simulink model "RB_KAIROS_ArmOnly"  (R2020b)
(part 10 of 17)

-t16229+t16408+t16412+t16445-q5d.*(t3933+t3938+t3951+t4005+t4112+t4113+t4134+t4154+t4229+t4246+t4307+t4325+t4454+t4458+t4463+t4523+t5038+t5089+t5148+t5157+t5202+t5353+t5381+t5473+t5512+t5567+t5662+t6241+t6342+t6347+t6369+t6562+t6652+t6708+t6712+t6714+t6723+t6752+t6768+t6769+t6919+t7058+t7523+t7596+t7597+t7609+t7679+t7722+t7742+t7760+t7905+t7947+t7988+t8037+t8059+t8078+t8196+t8425+t8443+t8446+t8662+t8680+t8736+t8748+t8773+t9037+t9039+t9294-t9304-t9351+t9539-t9543+t9575+t9587+t9607+t9692+t9697+t10370+t10493+t10503-t10576+t10667+t11245+t11261-t11450-t11460+t11665+t12004+t12081+t12087+t12282+t12284+(t5329.*(t2740+t3849+t3968+t3972-t5255+t17.*(t260+t468+t570+t2298).*7.35522e-1))./4.0+(t5441.*(-t1476-t1540+t2091+t2165+t2579+t8.*(t260+t468+t570+t2298)))./4.0+(t5345.*(-t3823+t3970+t5243+t9.*(t260+t468+t570+t2298).*7.35522e-1+t972.*(t71-t391)+t2777.*(t71-t391)))./4.0+(t6046.*(t1492+t2158+t2696-t4727))./4.0+(t4024.*(t3063+t3528+t3966-t5230))./4.0+(t3780.*(-t3045-t3218+t3458+t3539+t3878+t8.*(t260+t468+t570+t2298).*1.666555))./4.0+(t7796.*(t824+t2543+t2699+t2707-t4767+t17.*(t260+t468+t570+t2298)))./4.0+(t7797.*(-t2550+t2696+t2698+t4771+t9.*(t260+t468+t570+t2298)+t147.*(t71-t391)))./4.0)+q7d.*t16166-q3d.*t16340-q2d.*t16358+q4d.*(t3271+t3297+t3326+t3353+t3802+t3910+t3985+t4882+t5261+t5276+t5573+t5623+t6440+t6631+t6672+t6688+t6739+t6751+t8140+t8209+t8318+t13.*t35.*9.119126684115e-2+t13.*t42.*1.02650375589525e-1+t7.*t5928.*2.11820788799e-1+t15.*t5999.*2.11820788799e-1+t7.*t8044.*1.727815e-1+t15.*t8065.*1.727815e-1-(t4774.*t5331)./2.0-(t5443.*t7080)./2.0+(t4021.*t8709)./2.0-(t4024.*t8713)./2.0-(t6046.*t6744)./2.0+(t6069.*t6729)./2.0-(t3752.*t9104)./2.0+(t5696.*t10096)./2.0-(t5329.*t10753)./2.0-(t5345.*t10763)./2.0+(t8433.*t8477)./2.0-(t7796.*t9187)./2.0-(t7797.*t9197)./2.0+(t3424.*(t985+t3399-t13.*t42.*1.01140545e-1-t7.*t223.*5.034347249e-2))./2.0)-q6d.*(t4397+t4399+t4408+t4414+t4416+t4433+t4468+t4826+t4836+t4935+t4950-t5074+t5086+t5338+t5379+t5403+t5811+t5893+t6326+t6378+t6416+t6528+t6532+t6575+t7027+t7140+t7189+t7610+t7619+t8005+t8150+t8580+t8645+t8663+t8691+t8880+t9199+t9283+t9291+t9324+t9330+t9544+t9558-t9714+t9742-t9840+t10186+t10200+t10440+t10525-t10672+t10841+t10889-t10894+t10907+t11004+t11007+t11123+t11136+t11573+t11639+t11643+t12089+t12096+t8.*(t295-t13.*t42.*(3.3e+1./4.0e+2)).*5.01208083475e-2+t16.*(t295-t13.*t42.*(3.3e+1./4.0e+2)).*1.17633784675e-2),-t16190+t16359-t16361+t16365+phid.*(t2261+t2304+t2384+t3146+t3288+t3303+t3305+t3351+t3740+t4007+t4025+t4048+t4164+t4320+t4571+t4863+t4946+t4985+t5104+t5114+t5279+t5328+t5355+t5375+t5406+t5629+t5632+t5645+t5747+t5771+t5790+t5808+t5825+t5907+t5980+t6061+t6136+t6292+t6454+t6571+t6648+t6666+t6668+t6700+t6760+t6829+t6891+t6895+t6922+t7006+t7013+t7091+t7110+t7291+t7340+t7554+t7564+t7566+t7626+t7664+t7825+t7850+t7986+t8001+t8122+t8346+t8375+t8385+t8598+t8639+t8649+t8684+t8718+t8737+t8827+t8959+t9105+t10453+t10686-t10825-t10829-t10978+t10993-t11184+t11191+t11263+t11287-t11408-t11418+t11513-t11868+t11980+t12150+t12196+t12202+t12209-t12308-t12319-t12380-t12390-t12406+t12759+t12934+t13157-t13262-t13275+t13449+t13471-t13579-t13588+t13670+t13684+t13978+t14042-t14159+t14166+t14221-t14225+t14226+t14262-t14635-t14682-t14726-t14727-t14762-t14764+t15126+t15130+t15176+t15180+t15488+t15489+t15494+t15495+(t7987.*(t3418-t3879+t4324+t11855+t9.*(t71-t391).*4.5305948634e-2+t17.*(t426-t581).*7.35522e-1+t9.*(t9166-t11658).*7.35522e-1))./4.0+(t7130.*(t1589-t2213-t4346+t4355+t9454+t11863+t2772.*(t71-t391)+t2775.*(t71-t391)))./4.0+(t7982.*(t3423+t3845+t3888+t3925+t4339+t9.*(t210+t2107+t7423+t9121).*7.35522e-1+t17.*(t9166-t11658).*7.35522e-1))./4.0+(t9310.*(t249-t391.*(1.1e+1./1.25e+2)-t1912.*4.252e-3+t3505+t13496+t693.*(t71-t391)+t784.*(t71-t391)))./4.0+(t9887.*(t2091+t2497+t2579+t2680+t3516+t9.*(t210+t2107+t7423+t9121)+t17.*(t9166-t11658)))./4.0+(t9896.*(t1987-t2621+t3452+t11654+t9.*(t71-t391).*6.1597e-2+t17.*(t426-t581)+t9.*(t9166-t11658)))./4.0)-q6d.*t16216-q5d.*t16260+q3d.*t16327+q7d.*(t3995+t4013+t4190+t4197+t4271+t4313+t4437+t4467+t4543+t4560+t5106+t5166-t5688+t5906+t6001-t6439+t6487+t6491+t7633+t7758-t10457-t10565+t10573+t10755-t10760-t10844+t10845-t11160+t11236-t11240+(t5837.*(t395+t9.*(t48-t349)))./4.0+(t8477.*(-t2149+t2205+t693.*(t48-t349)+t784.*(t48-t349)))./4.0+(t5696.*(t3479-t3544+t2772.*(t48-t349)+t2775.*(t48-t349)))./4.0+(t15.*t16.*(-t2182+t2241+t696.*(t48-t349)+t891.*(t48-t349)))./4.0)+q4d.*((t5443.*(-t1272-t1479+t1647+t1848+t2236))./2.0+t5.*t6.*9.119126684115e-2+t5.*t14.*1.02650375589525e-1+t6.*t13.*1.644586079438601e-3-t13.*t14.*3.9053550262761e-3-(t7.*t4531)./2.0+(t15.*t4587)./2.0+t15.*t4837.*2.11820788799e-1-t7.*t4849.*2.11820788799e-1+(t370.*t4527)./2.0-(t404.*t4534)./2.0+(t7.*t6005)./2.0-(t404.*t5810)./2.0+(t540.*t5763)./2.0-t7.*t6552.*1.727815e-1+t15.*t6546.*1.727815e-1-(t325.*t6803)./2.0+(t229.*t6983)./2.0+(t3424.*t6092)./2.0+(t4265.*t5331)./2.0+(t5952.*t6046)./2.0-(t5951.*t6069)./2.0+(t4024.*t8062)./2.0-(t4021.*t8070)./2.0-(t5696.*t9310)./2.0+(t5329.*t9896)./2.0-(t5345.*t9887)./2.0-(t7130.*t8477)./2.0-(t7797.*t7982)./2.0+(t7796.*t7987)./2.0-(t5837.*(t106-t414))./2.0+(t3752.*(t2433+t2449-t3048-t3102+t3223+t3232))./2.0-(t14.*t43.*t3173)./2.0-(t14.*t37.*t3247)./2.0+(t6.*t13.*t3321)./2.0-(t14.*t43.*t4495)./2.0-(t15.*t16.*t6029)./2.0+(t8.*t15.*t6064)./2.0-(t15.*t16.*t6917)./2.0),-t16160-t16326+t16342+t16347+t16350+t16448+q7d.*t16137-q6d.*t16180-q5d.*t16236-q4d.*(t6.*(-3.9053550262761e-3)-t14.*1.644586079438601e-3-(t14.*t3321)./2.0+t7.*t4035.*2.11820788799e-1-t15.*t4064.*2.11820788799e-1-(t7.*t4383)./2.0+(t15.*t4451)./2.0+(t228.*t4534)./2.0-(t324.*t4527)./2.0+t7.*t5635.*1.727815e-1-t15.*t5646.*1.727815e-1+(t7.*t5845)./2.0+(t228.*t5810)./2.0-(t484.*t5837)./2.0+(t325.*t6637)./2.0+(t229.*t6758)./2.0+(t4024.*t6677)./2.0-(t4021.*t6681)./2.0+(t5443.*t5543)./2.0-(t5007.*t6069)./2.0+(t5050.*t6046)./2.0+(t3752.*t7676)./2.0-(t5696.*t8547)./2.0+(t6526.*t7797)./2.0+(t6540.*t7796)./2.0+(t5329.*t9048)./2.0+(t5345.*t9049)./2.0-(t6158.*t8477)./2.0+(t5763.*(t77-t390))./2.0+(t5331.*(t923-t1076))./2.0+(t3424.*(t2812-t2860))./2.0-(t6.*t15.*t3173)./2.0-(t6.*t7.*t3247)./2.0-(t6.*t15.*t4495)./2.0-(t8.*t15.*t5877)./2.0+(t15.*t16.*t5875)./2.0+(t15.*t16.*t6704)./2.0),q7d.*t16008+q6d.*t16115+q5d.*t16125,-t16126-t16238-t16262-t16297+t16310+t16313-t16427+q7d.*t16117+q6d.*t16151,-t16116+t16182+t16218+t16246+t16273+t16276+t16377+q7d.*t16112-q5d.*t16151,-t16009+t16139+t16154+t16165-t16193+t16264-q6d.*t16112-q5d.*t16117+yd.*(t8886+t8907+t11429+t11431-t13130-t13291+t14545+t14550-t14627-t14633+t14697+t14700-t14831-t14837),q4d.*(t8804+t8829+t9145+t9354-t10997-t10998+t11097+t11101+t11270+t11284+t11370+t11376-t11511-t11517+t11533+t11535-t11550+t11836+t11844-t12393-t12803-t12903-t13160+t13243+t13244+t13328+t13331-t13538+t13926+t13928+t14116+t14121+t14584+t14754+(t5441.*(t10158+t16.*(t4542-t6448)))./4.0+(t5213.*(t10403+t9.*(t10158+t16.*(t4542-t6448)).*7.35522e-1))./4.0+(t3266.*(t5110-t6808))./4.0+(t4879.*(t4542-t6448))./4.0+(t3780.*(t10384+t16.*(t4542-t6448).*1.666555))./4.0+(t7538.*(t10174+t9.*(t10158+t16.*(t4542-t6448))))./4.0)-phid.*(t7280+t7283+t8889+t8899-t10176+t10541+t11053+t11058+t12514+t12526+t12607+t12615+t12787+t12801+t14199+t14202+t14263+t14316+t14319+t14331+t14336+t14432+t14465+t14471+t14484+t14514+t14524+t14593+t14594+t14746+t14978+t14983+t15086+t15091+t15198+t15203+t15213+t15382+t15404+t15405+t15408+t15528+t15929+t15930+t15977+t15979+t15995+t15996+t16015+t16016)-q1d.*(t7280+t7283+t8889+t8899-t10176+t10541+t11053+t11058+t11833+t11839+t12036+t12141+t12153+t12179+t12192+t12420+t12423+t12429+t12492+t12514+t12526+t12607+t12615+t12676+t12677+t12787+t12801+t12835+t12947+t12951+t13058+t13477+t13488+t13574+t13671+t13683+t13940+t14207+t14465+t14471+t14514+t14524+t14728+t14729+t14979+t14982+t15133+t15135+t15288+t15290)-q7d.*t16183-q6d.*t16232-q3d.*t16331+q2d.*(t5581+t5592-t7358-t7366+t9411+t9440+t10019+t10409+t10660+t10693+t10828+t10837+t11089+t11096+t11471+t11489+t11697+t11733+t11737+t11939+t11962+t12056+t12061+t12070+t12242+t12244+t12264+t12412+t12612+t12613+t12716+t12851+t12868+t12950+t12967+t13153+t13222+t13240+t13424+t13431+t13598+t14014+t14414+t14415+t14701+t14706+t14912+t14915+t15118+t15119)+q5d.*(t15.*(t4540+t5.*(t2425-t2468)).*1.4653732538e-2-t2726.*(t4540+t5.*(t2425-t2468))-t22.*t10153.*1.7527158935e-2-t28.*t10153.*1.7527158935e-2-t2729.*t8077-t2744.*t8077+(t3249.*t10550)./2.0+(t4884.*t10147)./2.0+(t3738.*t13362)./2.0+(t3743.*t13357)./2.0+(t5433.*t13167)./2.0+(t5434.*t13172)./2.0-t16.*t3421.*t10153.*3.67761e-1-(t16.*t10153.*(t2904-t2927))./2.0),q5d.*(t6449.*(-1.4653732538e-2)-t8225.*1.4653732538e-2-t8229.*5.034347249e-2+t2726.*t6430+(t3249.*t10586)./2.0+(t4884.*t10164)./2.0+(t3738.*t13391)./2.0+(t3743.*t13387)./2.0+(t5433.*t13182)./2.0+(t5434.*t13189)./2.0+t22.*(t6452-t8229).*1.7527158935e-2+t28.*(t6452-t8229).*1.7527158935e-2+(t16.*(t2904-t2927).*(t6452-t8229))./2.0+t16.*t3421.*(t6452-t8229).*3.67761e-1)+q3d.*(t7300-t7310-t7313-t7315+t9405+t9475+t10265+t10291+t11036+t11045+t11172+t11183+t11259+t11260+t11330-t11394+t11405+t11413-t11559+t11588+t11595+t11681+t11789+t11845+t11914+t11918+t12318+t12470+t12949+t12957+t13059+t13062+t13289+t13658+t13668+t13672+t13757+t13764+t14117+t14127+t14392+t14406+t14704+t14705+t14906+t14911+t16.*(t6472-t9256).*4.38178973375e-3+t16.*(t6847-t9563).*2.62925e-3+(t3421.*(t6834-t9565))./4.0+((t2904-t2927).*(t6472-t9256))./4.0)+phid.*t16439-q7d.*t16186-q4d.*t16312+q1d.*(t7309+t7314+t8781+t8789+t10202+t10562+t11032+t11043-t12176-t12438+t12441+t12496+t12509+t12592+t12598-t12703+t12766+t12779-t12852-t12972+t13074+t13505-t13584+t13693+t13958+t14215+t14447+t14453+t14492+t14501-t14736-t14992+t15150+t15312+((t6806-t8574).*(t921+t1317-t5853))./4.0+((t6452-t8229).*(t2810+t2988-t7937))./4.0+(t14213.*(t2740+t3849+t3968+t3972-t5255+t17.*(t260+t468+t570+t2298).*7.35522e-1))./4.0+(t13189.*(t3418-t3879+t4324-t5228+t5802+t9.*(t71-t391).*4.5305948634e-2+t17.*(t426-t581).*7.35522e-1))./4.0+(t13391.*(t1987-t2621+t3452-t4730+t5359+t9.*(t71-t391).*6.1597e-2+t17.*(t426-t581)))./4.0+(t12508.*(t1492+t2158+t2696-t4727))./4.0+(t12307.*(t3063+t3528+t3966-t5230))./4.0+(t10577.*(t495+t572+t1838+t2069+t2107))./4.0+(t10164.*(t2437+t2648+t3129+t3384+t3574))./4.0+(t5853.*(t6806-t8574))./4.0+(t6535.*(t6801-t8594))./4.0+(t7937.*(t6452-t8229))./4.0+(t8791.*(t6452-t8229))./4.0+(t14299.*(t824+t2543+t2699+t2707-t4767+t17.*(t260+t468+t570+t2298)))./4.0+t16.*t8227.*(t6452-t8229).*4.1663875e-1+(t16.*t9744.*(t6452-t8229))./4.0)+q6d.*(t10652+t11056+t11064+t12702+t12707+t12786+t12797+t12800+t12809+t12929+t12935+t13402-t13405+t13520-t13533+t14472+t14475+t14521+t14525+t16.*(t6452-t8229).*5.01208083475e-2+t16.*t3489.*(t6452-t8229).*1.838805e-1+(t16.*t5365.*(t6452-t8229))./4.0)-q2d.*(t5624+t5630+t7408+t7426+t9491+t9500+t10037+t10422+t10741+t10752+t10866+t10874+t11146+t11167-t11488+t11503+t11719+t11754-t11960+t11981+t12064+t12263+t12280+t12728+t12906+t12914+t13015+t13029-t13245-t13272-t13439-t13452-t13602-t14026+t14428+t14430+t14717+t14721+t14931-t14936+t15125-t15129+(t5634.*(t6806-t8574))./4.0+(t8050.*(t6452-t8229))./4.0+t16.*t7079.*(t6452-t8229).*4.1663875e-1+t8.*t7116.*(t6452-t8229).*4.1663875e-1+t16.*t8191.*(t6452-t8229).*1.838805e-1+(t8.*t9112.*(t6452-t8229))./4.0+(t16.*t9110.*(t6452-t8229))./4.0+(t16.*t10141.*(t6452-t8229))./4.0),t16353+t16436+q6d.*t16356-q4d.*t16425-q3d.*t16428-q2d.*t16440+q7d.*(-t4652-t4658+t4757+t4825+t5253+t5305+t5766+t5791+t7139+t7199+t7204+t8632+t8677+t8904+t9266+t12008+t12014+t12018+t14555+t14872+t15553+t15555+t15600+t15602+t15607+t15609+t15671+t15672+t8.*t11672.*3.867742437e-3+t2963.*(t71-t391)+t3167.*(t71-t391)+t4080.*(t71-t391)+t4130.*(t71-t391))+q5d.*(t4111+t4141+t4250+t4312-t4336+t4366+t4405-t4444+t5094+t5505-t5528-t6281+t6297+t7401.*1.4653732538e-2+t7552+t16.*(t1292+t2073+t2694+t11671).*8.7635794675e-3-(t5433.*(-t2550+t2696+t2698+t11659+t8.*t11672+t147.*(t71-t391)))./2.0-(t3743.*(-t3823+t3970+t11861+t8.*t11864+t972.*(t71-t391)+t2777.*(t71-t391)))./2.0-t2726.*t7344-t8.*t12392.*8.7635794675e-3-t8.*t12792.*5.2585e-3-(t3249.*t12898)./2.0+(t3421.*t13578)./2.0-(t4884.*t12266)./2.0-(t3738.*t15088)./2.0-(t5434.*t14770)./2.0+t3620.*(t71-t391)+(t12866.*(t2904-t2927))./2.0+t2729.*(-t211+t5081+t7275)+t2744.*(-t211+t5081+t7275)+t16.*(t3116+t3486+t3963+t11671.*1.666555).*5.2585e-3+(t16.*t17.*(t578.*4.28e-4+t2566-t2597+t905.*(t71-t391)+t1021.*(t71-t391)))./2.0+(t9.*t16.*(t578.*1.2516e-2+t2492-t2628+t2673+t1129.*(t71-t391)))./2.0)+q1d.*(t5882+t5909+t5994+t6543+t6782+t6854+t7120+t7165+t7889+t7975+t7991+t8042+t8045+t8246+t8535+t8621+t8894+t9066+t9109+t9364+t9383-t9580-t10145+t11824+t11834-t12218-t12604+t13210+t13216+t13321+t13323+t13464+t13483+t13613+t13614-t13817+t13833+t13834-t14019-t14020-t14105-t14106+t14637+t14692+t14806+t14903+t15020+t15022+t15067+t15071+t15367+t15396+t15650+t15666+t15836-t15838-t15844+t15845+(t9744.*(t1292+t2073+t2694+t11671))./4.0+((-t3045+t3539+t14113).*(t1492+t2158+t2696-t4727))./4.0+((-t1476+t2165+t13876).*(t3063+t3528+t3966-t5230))./4.0+((t2810+t2988-t12589).*(t495+t572+t1838+t2069+t2107))./4.0+((t921+t1317-t5853).*(t3129+t3384+t3574+t7846+t9332))./4.0+(t11470.*(-t2550+t2696+t2698+t11659+t8.*t11672+t147.*(t71-t391)))./4.0+(t10149.*(-t3823+t3970+t11861+t8.*t11864+t972.*(t71-t391)+t2777.*(t71-t391)))./4.0+(t12792.*(-t1476-t1540+t2091+t2165+t2579+t8.*(t260+t468+t570+t2298)))./4.0+(t12385.*(t2437+t2648+t3129+t3384+t3574))./4.0+(t12392.*(-t3045-t3218+t3458+t3539+t3878+t8.*(t260+t468+t570+t2298).*1.666555))./4.0+(t8227.*(t3116+t3486+t3963+t11671.*1.666555))./4.0)+yd.*(t7328+t7338+t8774+t8795+t10202+t10562+t11039+t11047+t12499+t12504+t12595+t12596+t12771+t12783+t14211+t14214+t14269+t14328+t14335+t14342+t14344+t14437+t14448+t14451+t14490+t14494+t14498+t14614+t14615+t14751+t14988+t14991+t15105+t15110+t15207+t15208+t15224+t15392+t15413+t15415+t15416+t15532+t15942+t15943+t15981+t15986+t16004+t16007+t16023+t16027),-t16207-t16368-t16433-q4d.*(t3933+t3938+t3951+t4005+t4112+t4113+t4134+t4154+t4229+t4246+t4307+t4325+t4454+t4458+t4463+t4523+t5038+t5089+t5148+t5157+t5202+t5353+t5381+t5473+t5512+t5567+t5662+t6241+t6342+t6347+t6369+t6562+t6652+t6708+t6712+t6714+t6723+t6752+t6768+t6769+t6919+t7058+t7523+t7596+t7597+t7609+t7679+t7722+t7742+t7760+t7905+t7947+t7988+t8037+t8059+t8078+t8196+t8425+t8443+t8446+t8662+t8680+t8736+t8748+t8773+t9037+t9039+t9294-t9304-t9351+t9539-t9543+t9575+t9587+t9607+t9692+t9697+t10370+t10493+t10503-t10576+t10667+t11245+t11261-t11450-t11460+t11665+t12004+t12081+t12087+t12282+t12284+(t5329.*(t2740+t3849+t3968+t3972-t5255+t17.*(t260+t468+t570+t2298).*7.35522e-1))./4.0+(t5441.*(-t1476-t1540+t2091+t2165+t2579+t8.*(t260+t468+t570+t2298)))./4.0+(t5345.*(-t3823+t3970+t5243+t9.*(t260+t468+t570+t2298).*7.35522e-1+t972.*(t71-t391)+t2777.*(t71-t391)))./4.0+(t6046.*(t1492+t2158+t2696-t4727))./4.0+(t4024.*(t3063+t3528+t3966-t5230))./4.0+(t3780.*(-t3045-t3218+t3458+t3539+t3878+t8.*(t260+t468+t570+t2298).*1.666555))./4.0+(t7796.*(t824+t2543+t2699+t2707-t4767+t17.*(t260+t468+t570+t2298)))./4.0+(t7797.*(-t2550+t2696+t2698+t4771+t9.*(t260+t468+t570+t2298)+t147.*(t71-t391)))./4.0)+q6d.*t16224-q3d.*t16316-q2d.*t16328+q7d.*(-t4652-t4658+t4757+t4825+t5253+t5305+t5687-t5698+t5766+t5791+t7139+t7199+t7204+t8632+t8677+t8904+t9266+t10330+t10589+t10591+t10853+t10861+t10967+t10977+t11455+t11823+t11832+t9.*(t260+t468+t570+t2298).*3.867742437e-3+t17.*(t260+t468+t570+t2298).*1.563719772e-3+t2963.*(t71-t391)+t3167.*(t71-t391)+t4080.*(t71-t391)+t4130.*(t71-t391))+yd.*(t7328+t7338+t8774+t8795+t10202+t10562+t11039+t11047-t12176-t12438+t12441+t12499+t12504+t12595+t12596-t12703+t12771+t12783-t12852-t12972+t13074+t13505-t13584+t13693+t13958+t14215+t14448+t14451+t14494+t14498-t14736-t14992+t15150+t15312+((t6806-t8574).*(t921+t1317-t5853))./4.0+((t6452-t8229).*(t2810+t2988-t7937))./4.0+(t14213.*(t2740+t3849+t3968+t3972-t5255+t17.*(t260+t468+t570+t2298).*7.35522e-1))./4.0+(t13189.*(t3418-t3879+t4324-t5228+t5802+t9.*(t71-t391).*4.5305948634e-2+t17.*(t426-t581).*7.35522e-1))./4.0+(t13391.*(t1987-t2621+t3452-t4730+t5359+t9.*(t71-t391).*6.1597e-2+t17.*(t426-t581)))./4.0+(t12508.*(t1492+t2158+t2696-t4727))./4.0+(t12307.*(t3063+t3528+t3966-t5230))./4.0+(t10577.*(t495+t572+t1838+t2069+t2107))./4.0+(t10164.*(t2437+t2648+t3129+t3384+t3574))./4.0+(t5853.*(t6806-t8574))./4.0+(t6535.*(t6801-t8594))./4.0+(t7937.*(t6452-t8229))./4.0+(t8791.*(t6452-t8229))./4.0+(t14299.*(t824+t2543+t2699+t2707-t4767+t17.*(t260+t468+t570+t2298)))./4.0+t16.*t8227.*(t6452-t8229).*4.1663875e-1+(t16.*t9744.*(t6452-t8229))./4.0)+q5d.*(t464.*(-5.034347249e-2)+t468.*1.4653732538e-2+t570.*1.4653732538e-2+t572.*5.034347249e-2+t4111+t4141+t4250+t4312-t4336+t4366+t4405-t4444+t5094+t5505-t5528-t6281+t6297+t7552-(t3738.*(t2740+t3849+t3968+t3972-t5255+t17.*(t260+t468+t570+t2298).*7.35522e-1))./2.0-(t3743.*(-t3823+t3970+t5243+t9.*(t260+t468+t570+t2298).*7.35522e-1+t972.*(t71-t391)+t2777.*(t71-t391)))./2.0+t16.*t6995.*8.7635794675e-3+t16.*t8600.*5.2585e-3-(t4884.*t6535)./2.0-(t3249.*t8791)./2.0+(t3421.*t10240)./2.0-t8.*(t1492+t2158+t2696-t4727).*8.7635794675e-3-t8.*(t3063+t3528+t3966-t5230).*5.2585e-3+t3620.*(t71-t391)+(t8693.*(t2904-t2927))./2.0-(t5434.*(t824+t2543+t2699+t2707-t4767+t17.*(t260+t468+t570+t2298)))./2.0-(t5433.*(-t2550+t2696+t2698+t4771+t9.*(t260+t468+t570+t2298)+t147.*(t71-t391)))./2.0+(t16.*t17.*(t578.*4.28e-4+t2566-t2597+t905.*(t71-t391)+t1021.*(t71-t391)))./2.0+(t9.*t16.*(t578.*1.2516e-2+t2492-t2628+t2673+t1129.*(t71-t391)))./2.0),t16176+t16339+t16344+t16442+q1d.*(t3806+t3818+t3974+t3983+t4108+t4155+t4171+t4184+t4245+t4316+t4343+t4431+t4439+t4766+t4803+t5368+t5520+t5548+t5627+t5717+t5768+t5770+t5792+t5799+t6059+t6157+t6266+t6389+t6426+t6429+t6557+t6564+t6945+t7035+t7143+t7203+t7211+t7375+t7592+t7616+t7706+t7711+t7812+t7816+t7843+t7906+t7924+t8200+t8257+t8359+t8409+t8611+t8625+t8664+t8726+t8901+t8924+t8965+t9004+t9192+t9308-t9352+t9672+t9676+t9883+t9900+t9927+t9937+t9938-t9969+t9990+t10015+t10281+t10347+t10366+t10516+t10717-t10751+t10788-t10805+t11029-t11060+t11104-t11133+t11302+t11310+t11411+t12001+t12003-t12356+t12404-t12460+t12490+t12812+t12813+t12938+t12940+(t8979.*(t2740+t3849+t3968+t3972-t5255+t17.*(t260+t468+t570+t2298).*7.35522e-1))./4.0+(t7646.*(-t1476-t1540+t2091+t2165+t2579+t8.*(t260+t468+t570+t2298)))./4.0+(t8981.*(-t3823+t3970+t5243+t9.*(t260+t468+t570+t2298).*7.35522e-1+t972.*(t71-t391)+t2777.*(t71-t391)))./4.0+(t9112.*(t1492+t2158+t2696-t4727))./4.0+(t7116.*(t3063+t3528+t3966-t5230))./4.0+(t6014.*(-t3045-t3218+t3458+t3539+t3878+t8.*(t260+t468+t570+t2298).*1.666555))./4.0+(t10468.*(t824+t2543+t2699+t2707-t4767+t17.*(t260+t468+t570+t2298)))./4.0+(t10469.*(-t2550+t2696+t2698+t4771+t9.*(t260+t468+t570+t2298)+t147.*(t71-t391)))./4.0)+q7d.*t16141-q6d.*t16198-q4d.*t16260+q3d.*t16285+q5d.*(t31.*1.026787777028894e-3+t36.*1.716784138406187e-2+t37.*1.590853730684e-2-t43.*4.630579482008e-3-t59.*2.16405205209813e-3+t72.*4.600245517563106e-3+t492.*5.034347249e-2-t496.*1.4653732538e-2+t507.*1.4653732538e-2+t509.*5.034347249e-2+t321.*t3620+(t605.*t4410)./2.0-(t754.*t4515)./2.0+(t8.*t5644)./2.0-(t16.*t5640)./2.0+t16.*t5929.*8.7635794675e-3-t8.*t6014.*8.7635794675e-3+(t8.*t6634)./2.0+t16.*t7622.*5.2585e-3-t8.*t7646.*5.2585e-3-(t4884.*t5523)./2.0+(t3421.*t9505)./2.0-(t5434.*t7799)./2.0-(t3738.*t9537)./2.0-(t3743.*t9538)./2.0-(t3249.*(t917-t1669+t2469+t2475+t3495+t3591))./2.0-(t225.*(t733-t806))./2.0+(t7336.*(t2904-t2927))./2.0-(t5433.*(t2056+t2203+t2351+t3433+t3503+t16.*t389.*(1.1e+1./1.25e+2)))./2.0-(t16.*t321.*t3296)./2.0-(t16.*t321.*t4477)./2.0+(t9.*t16.*t6573)./2.0+(t16.*t17.*t6629)./2.0),t16286+t16318+t16333+t16336+t16430-q7d.*t16127-q4d.*t16236-q6d.*(t3683-t3711+t3905+t3992+t3998+t4004+t4012+t4059-t4070-t4138-t4151-t4177+t4852+t4878+t4885+t4951+t4976+t5059+t5370+t5399+t5595+t5618+t5654+t5697+t5735+t5948+t5991+t6006-t6089+t6217+t6218+t6488+t6489+t6703+t6730+t6819-t6959-t6979+t7019+t7191+t7419+t7420+t7425+t7630+t8036+t8288+t8290+t8308-t8439-t8783-t8787+t8930+t8943+t9010+t9017+t9019-t9164+t9251+t9923+t9930+(t371.*(t689-t740))./4.0)+q3d.*(t3633+t3726-t3746+t4595-t4642+t4830-t4966+t4993-t5977+t6037-t6056-t6130-t6131+t6269-t6334-t6679+t6697+t6774+t6978-t7060-t7170+t7175-t8168+t8180-t8511+t8521-t8809-t9232+t10278+t10279+t10520-t10540+t10771-t10776+(t5990.*(t79-t358))./2.0)-q5d.*(t7.*4.153336480425e-3-t15.*1.208932934385e-3-t421.*5.034347249e-2+t422.*1.4653732538e-2+t7.*t14.*2.16405205209813e-3-t14.*t15.*4.600245517563106e-3+t16.*t4489.*8.7635794675e-3+t8.*t4509.*8.7635794675e-3-(t8.*t4711)./2.0+(t16.*t4726)./2.0-(t405.*t4410)./2.0+(t371.*t4515)./2.0+t8.*t5912.*5.2585e-3+t16.*t5919.*5.2585e-3-(t8.*t5981)./2.0+(t4453.*t4884)./2.0+(t3249.*t6385)./2.0+(t5434.*t6016)./2.0-(t5433.*t6038)./2.0-(t3421.*t8497)./2.0+(t3738.*t8460)./2.0-(t3743.*t8464)./2.0-(t6096.*(t2904-t2927))./2.0-(t15.*t44.*t3296)./2.0+(t15.*t39.*t3307)./2.0-(t15.*t44.*t4477)./2.0+(t9.*t16.*t5888)./2.0+(t16.*t17.*t5990)./2.0+(t7.*t14.*(t733-t806))./2.0),t16126+t16238+t16262+t16297+t16427+xd.*(t8808+t8820+t9138+t9343-t10997-t10998+t11097+t11101+t11270+t11284+t11360+t11384-t11511-t11517+t11528+t11542-t11550+t11840+t11853-t12393-t12803-t12903-t13160+t13238+t13251+t13324+t13334-t13538+t13926+t13928+t14116+t14121+t14584+t14754+(t5441.*(t10158+t16.*(t4542-t6448)))./4.0+(t5213.*(t10403+t9.*(t10158+t16.*(t4542-t6448)).*7.35522e-1))./4.0+(t3266.*(t5110-t6808))./4.0+(t4879.*(t4542-t6448))./4.0+(t3780.*(t10384+t16.*(t4542-t6448).*1.666555))./4.0+(t7538.*(t10174+t9.*(t10158+t16.*(t4542-t6448))))./4.0)+q7d.*t16119+q6d.*t16150+yd.*(t8846+t8856+t9151-t9348+t9369-t9396+t11122+t11125+t11303+t11314+t11427+t11445+t11598+t11610+t11880+t11894-t12825-t12840-t12922-t12932-t13174+t13287+t13295+t13366+t13378-t13555+t13962+t13965+t14139+t14145+t14595-t14596+t14780-t14787+t8.*t4024.*(t6452-t8229).*4.1663875e-1+t16.*t4021.*(t6452-t8229).*4.1663875e-1+t16.*t5696.*(t6452-t8229).*1.838805e-1+(t8.*t6046.*(t6452-t8229))./4.0+(t16.*t6069.*(t6452-t8229))./4.0+(t16.*t8477.*(t6452-t8229))./4.0)+q5d.*(t7.*(-1.026787777028894e-3)-t15.*1.716784138406187e-2+t7.*t3588-t16.*t3732.*8.7635794675e-3+t8.*t3780.*8.7635794675e-3-(t8.*t4532)./2.0+(t16.*t4526)./2.0+t7.*t4617-(t230.*t4410)./2.0+(t326.*t4515)./2.0-t16.*t5430.*5.2585e-3+t8.*t5441.*5.2585e-3-(t8.*t5821)./2.0+(t3771.*t4884)./2.0+(t3249.*t5442)./2.0+(t5213.*t5434)./2.0+(t5217.*t5433)./2.0+(t3738.*t7538)./2.0+(t3743.*t7540)./2.0-(t3421.*t7980)./2.0+(t15.*(t733-t806))./2.0-(t5524.*(t2904-t2927))./2.0-(t7.*t8.*t3307)./2.0-(t9.*t16.*t5761)./2.0-(t16.*t17.*t5834)./2.0),-q7d.*t14553+q6d.*t15781,-t15782-t16153+t16168+t16199+t16223-t16231+t16355+q7d.*t15892+yd.*(t10652+t11059+t11068+t12698+t12710+t12791+t12794+t12804+t12806+t12928+t12936+t13402-t13405+t13520-t13533+t14470+t14477+t14518+t14527+t16.*(t6452-t8229).*5.01208083475e-2+t16.*t3489.*(t6452-t8229).*1.838805e-1+(t16.*t5365.*(t6452-t8229))./4.0),t14558-t16118-t16129+t16142-t16185-t16188-q6d.*t15892+phid.*(-t4652-t4658+t4757+t4840+t5267+t5296+t5773+t5803+t7148+t7195+t7207+t8626+t8682+t8881+t9257+t12008+t12014+t12018+t14549+t14869+t15554+t15558+t15597+t15601+t15608+t15610+t15669+t15670+t8.*t11672.*3.867742437e-3+t2963.*(t71-t391)+t3167.*(t71-t391)+t4080.*(t71-t391)+t4130.*(t71-t391))+q1d.*(-t4652-t4658+t4757+t4840+t5267+t5296+t5687-t5698+t5773+t5803+t7148+t7195+t7207+t8626+t8682+t8881+t9257+t10321+t10578+t10599+t10855+t10857+t10965+t10979+t11452+t11827+t11828+t9.*(t260+t468+t570+t2298).*3.867742437e-3+t17.*(t260+t468+t570+t2298).*1.563719772e-3+t2963.*(t71-t391)+t3167.*(t71-t391)+t4080.*(t71-t391)+t4130.*(t71-t391)),q6d.*((t5365.*(t10158+t16.*(t4542-t6448)))./2.0+t23.*t12279.*4.5305948634e-2+t29.*t12279.*4.5305948634e-2+t2766.*t10147+t2782.*t10147+t16.*(t4542-t6448).*1.00241616695e-1-t2762.*(t4542-t6448)+(t3489.*(t10378+t16.*(t4542-t6448).*7.35522e-1))./2.0)-phid.*t16401-q5d.*t16232+q4d.*t16274-q3d.*t16287-q2d.*t16302-q1d.*t16319-q7d.*(t12494+t12498-t12750+(t12484.*(t701-t775))./4.0),q2d.*(t8957+t8962+t11170+t11346+t11723+t12027+t12567+t12569+t12682+t12690+t13257+t13258+t13361+t13443+t13450+t13547+t13549+t13581+t13820+t13917+t13922+t13929+t13938+t14183+t14256+t14259+t14875+t14876+t15011+t15015-t8.*(t30.*(t2425-t2468)+t68.*(t2425-t2468)).*5.01208083475e-2-t16.*(t30.*(t2425-t2468)+t68.*(t2425-t2468)).*1.17633784675e-2)+q3d.*(t7311+t7321+t9797+t9809+t11884+t11990-t12944+t12959-t13045-t13054+t13064+t13106-t13110-t13147+t13274-t13280-t13319+t13352-t13367+t13389+t13397+t13498+t13509-t13713+t13972-t13977-t14671+t14680-t14846+t14848+(t5275.*(t6801-t8594))./4.0+(t6969.*(t6452-t8229))./4.0)+phid.*t16406+q1d.*t16324-q7d.*(t12511+t12518-t12774+(t12500.*(t701-t775))./4.0)-q4d.*(t8890-t8893-t8900-t8911+t11074+t11085+t12723+t12726+t12820+t12829+t12874+t12877+t12896-t13006+t13021+t13034+t13084+t13099+t13103-t13132+t13194+t13495+t13502+t13659+t14528+t14538+t14638+t14639+t17.*(t8221-t11008).*1.13264871585e-2+t17.*(t8583-t11188).*1.539925e-2+(t3489.*(t8582-t8586))./4.0+(t5365.*(t8219-t8226))./4.0)+q5d.*(t10652+t11056+t11064+t12702+t12707+t12786+t12797+t12800+t12809+t12929+t12935+t13402-t13405+t13520-t13533+t14472+t14475+t14521+t14525+t16.*(t6452-t8229).*5.01208083475e-2+t16.*t3489.*(t6452-t8229).*1.838805e-1+(t16.*t5365.*(t6452-t8229))./4.0)+q6d.*(t8192.*(-1.00241616695e-1)+t2762.*(t6460-t35.*(t2425-t2468))+t23.*t12296.*4.5305948634e-2+t29.*t12296.*4.5305948634e-2+t2766.*t10164+t2782.*t10164-(t3489.*t12506)./2.0-(t5365.*t12307)./2.0),-t16315+t16403-q2d.*(t4232+t4409+t4413+t4417+t4698+t4715+t4813+t5184+t5238+t6375-t6485-t6572+t6608+t7114-t7243-t7432+t7549-t7640+t7911+t7925-t8134+t8165+t8268+t8528+t8542+t8579+t8659+t8758+t8801+t8885-t10120+t10287+t10300-t10856+t13634+t13698+t14009+t14077+t14644+t14646-t14650-t14652+t14672+t14675-t14742-t14743+t14759+t14765+t14947+t14962+t14965+t15131-t15197-t15199-t15267-t15268+t15769-t15776+t15787-t15792+(t6041.*(t1918+t9.*(t71-t391)))./4.0+(t10141.*(t3625+t3660+t9166-t11658))./4.0+(t8191.*(t4401+t4424+t9457-t11860))./4.0+(t5586.*(t71-t391))./4.0+(t5582.*(t348-t525))./4.0+(t6720.*(t348-t525))./4.0+((t348-t525).*(t1254+t1943+t9.*t439.*1.196e-3+t439.*t1083))./4.0)+q7d.*t16255+q5d.*t16356-q3d.*t16379-q4d.*t16378-q1d.*t16385+yd.*(-t10580+t10587+t11945+t12174-t12785-t12888-t14289-t14345+t15521+t15522+t15544+t15546+t15547+t15578+t15583+t15594+t15632+t15639+t15644+t15740+t15872+t15873+t15887+t15888+t15911+t15912+t15970+t15972+t9.*(t10403+t9.*(t10158+t16.*(t4542-t6448)).*7.35522e-1).*1.539925e-2+t8.*(t4542-t6448).*5.01208083475e-2+t16.*(t4542-t6448).*1.17633784675e-2+t9.*(t10174+t9.*(t10158+t16.*(t4542-t6448))).*1.13264871585e-2)-q6d.*(t4318+t4364-t4623+t4684+t4695+t6990+t7078-t9166.*1.00241616695e-1+t2762.*t9156-t9.*t14161.*2.2652974317e-2+t17.*t14156.*2.2652974317e-2+t2766.*t11633+t2782.*t11633-t9.*t14413.*3.07985e-2+t17.*t14411.*3.07985e-2-(t5365.*(t3625+t3660+t9166-t11658))./2.0-(t3489.*(t4401+t4424+t9457-t11860))./2.0+t3398.*(t348-t525)+t3550.*(t348-t525)),-t16171+t16321-t16387+q7d.*t16146+q5d.*t16224-q3d.*t16249-q2d.*(t4225+t4232+t4268+t4409+t4413+t4417+t4698+t4715+t4813+t5184+t5238+t5651+t5684+t6375-t6485-t6572+t6608+t7114-t7243-t7432+t7549-t7640+t7911+t7925-t8134+t8165+t8268+t8579+t8659+t8758+t8801+t8885-t10120+t10421+t10482+t10638+t10645+t10732-t10749+t10789-t10856+t11049-t11054+t11109+t11126+t11423+t11487+t11691+t11718+t11725+t12090+t12248-t12431-t12432-t12572-t12585-t12594-t12599-t12815-t12821+(t6041.*(t1918+t9.*(t71-t391)))./4.0+(t7613.*(-t1476-t1540+t2091+t2165+t2579+t8.*(t260+t468+t570+t2298)))./4.0+(t5586.*(t71-t391))./4.0+(t5582.*(t348-t525))./4.0+(t6720.*(t348-t525))./4.0+((t348-t525).*(t1254+t1943+t9.*t439.*1.196e-3+t439.*t1083))./4.0+(t5923.*(-t3045-t3218+t3458+t3539+t3878+t8.*(t260+t468+t570+t2298).*1.666555))./4.0)+yd.*(-t10580+t10587+t11945+t12174-t12785-t12888+t13485+t13494+t13662+t13685+t13690+t13830+t13831+t13870+t14072+t14081+t14093+t14243+t14245-t14289-t14345+t14393+t14575+t14579+t15059+t15062+t15204+t15206+t9.*(t10403+t9.*(t10158+t16.*(t4542-t6448)).*7.35522e-1).*1.539925e-2+t8.*(t4542-t6448).*5.01208083475e-2+t16.*(t4542-t6448).*1.17633784675e-2+t9.*(t10174+t9.*(t10158+t16.*(t4542-t6448))).*1.13264871585e-2)-q6d.*(t1510.*2.3526756935e-2-t1540.*1.00241616695e-1+t4318+t4364-t4623+t4684+t4695+t6990+t7078+t2766.*(t260+t468+t570+t2298)+t2782.*(t260+t468+t570+t2298)+t17.*t8725.*2.2652974317e-2-t9.*t8743.*2.2652974317e-2-t9.*t9926.*3.07985e-2+t17.*t9922.*3.07985e-2-(t3489.*t9028)./2.0-(t5365.*t7654)./2.0+t3398.*(t348-t525)+t3550.*(t348-t525))-q4d.*(t4397+t4399+t4408+t4414+t4416+t4433+t4468+t4826+t4836+t4935+t4950-t5074+t5086+t5338+t5379+t5403+t5811+t5893+t6326+t6378+t6416+t6528+t6532+t6575+t7027+t7140+t7189+t7610+t7619+t8005+t8150+t8580+t8645+t8663+t8691+t8880+t9199+t9283+t9291+t9324+t9330+t9544+t9558-t9714+t9742-t9840+t10186+t10200+t10440+t10525-t10672+t10841+t10889-t10894+t10907+t11004+t11007+t11123+t11136+t11573+t11639+t11643+t12089+t12096+t8.*(t295-t13.*t42.*(3.3e+1./4.0e+2)).*5.01208083475e-2+t16.*(t295-t13.*t42.*(3.3e+1./4.0e+2)).*1.17633784675e-2),t16149+t16267+t16304+t16396-q6d.*(t48.*(-9.3569097314605e-5)-t75.*1.037589172186849e-4+t349.*9.3569097314605e-5-t355.*1.037589172186849e-4+t620.*2.3526756935e-2-t624.*1.00241616695e-1+t9.*(t1468-t1988-t2498+t4565+t17.*(t208-t427)).*2.2652974317e-2+(t17.*t5955)./2.0-(t9.*t6041)./2.0+t2766.*t3330+t2782.*t3330+t17.*t7348.*2.2652974317e-2+t17.*t9050.*3.07985e-2-(t3286.*(t48-t349))./2.0+t9.*(t3085-t3419-t3773+t5128+t17.*(t208-t427).*7.35522e-1).*3.07985e-2-(t3489.*(t2752+t3814-t4385-t9.*t439.*3.127439544e-3))./2.0-(t5365.*(t624+t2511-t3502-t9.*t439.*4.252e-3))./2.0-(t9.*t439.*t3239)./2.0+(t17.*t439.*(t689-t740))./2.0)-q5d.*t16198-q4d.*t16216+q3d.*t16241-q7d.*(t4201+t4248-t4443-t4577+t4593+t4675+t4706+t4741+t4788-t5568+t5585+t6270+t6382+t7494+t7575+t8573+t8704+t8708+t8825+t9404+t9434+t9443+t9680+t9681+t10696+t10728+t10730+t9.*(t208-t427).*3.867742437e-3+t17.*(t208-t427).*1.563719772e-3)+yd.*(t8952-t11170+t11723+t12027-t12690+t13257+t13258+t13361+t13443+t13450+t13547+t13549+t13581+t13820+t13917+t13922+t13929+t13938+t14183+t14256+t14259+t14875+t14876+t15011+t15015+t9.*(t9.*(t16.*(t30.*(t2425-t2468)+t68.*(t2425-t2468))+t8.*(t7.*(t4650+t34.*(t2425-t2468))+t47.*(t2425-t2468)))+t17.*(t4654+t15.*(t4650+t34.*(t2425-t2468)))).*1.13264871585e-2+t8.*(t30.*(t2425-t2468)+t68.*(t2425-t2468)).*5.01208083475e-2+t16.*(t30.*(t2425-t2468)+t68.*(t2425-t2468)).*1.17633784675e-2+t8.*(t7.*(t4650+t34.*(t2425-t2468))+t47.*(t2425-t2468)).*1.17633784675e-2+(t5365.*(t8315+t8.*(t30.*(t2425-t2468)+t68.*(t2425-t2468))))./4.0+t17.*(t8329+t17.*(t16.*(t30.*(t2425-t2468)+t68.*(t2425-t2468))+t8.*(t7.*(t4650+t34.*(t2425-t2468))+t47.*(t2425-t2468)))).*1.13264871585e-2+t9.*(t9.*(t16.*(t30.*(t2425-t2468)+t68.*(t2425-t2468))+t8.*(t7.*(t4650+t34.*(t2425-t2468))+t47.*(t2425-t2468))).*7.35522e-1+t17.*(t4654+t15.*(t4650+t34.*(t2425-t2468))).*7.35522e-1).*1.539925e-2),-t16131-t16251-t16289-t16292-t16381-q6d.*(t32.*1.037589172186849e-4+t38.*9.3569097314605e-5+t63.*9.3569097314605e-5-t76.*1.037589172186849e-4+t598.*2.3526756935e-2+t622.*1.00241616695e-1+(t227.*t3286)./2.0+t323.*t3398+t323.*t3550+(t17.*t5561)./2.0+(t9.*t5609)./2.0+t17.*t5760.*2.2652974317e-2-t9.*t5782.*2.2652974317e-2+t17.*t7901.*3.07985e-2-t9.*t7913.*3.07985e-2+(t3489.*t6304)./2.0+(t4964.*t5365)./2.0)+q2d.*(-t4065-t4081-t4136-t4175+t4180-t4234-t4376-t4419-t4974+t4990+t5545+t5691+t5718+t5745+t5865+t5867+t5941+t6282+t6348+t6352+t6388+t6398+t6412+t6464+t7033+t7076+t7086+t7122+t7167+t7455-t7537+t7669+t7698+t7782+t9221+t9235+t9243+t9246+t9286+t9295+t9329-t9486-t9489-t9612+t9660+t9807+t10027+t10035+t10077+t10126+t10458+t10492-t10680-t10745-t10748+t10935+t10958+t11034+t11313+t11318+t11337+t11357+t11680+t11684+(t1837.*(t689-t740))./4.0+(t3286.*(t60-t394))./4.0+(t3239.*(t357-t519))./4.0)+q7d.*t16120-q4d.*t16180-q5d.*(t3683-t3711+t3905+t3992+t3998+t4004+t4012+t4059-t4070-t4138-t4151-t4177+t4852+t4878+t4885+t4951+t4976+t5059+t5370+t5399+t5595+t5618+t5654+t5697+t5735+t5948+t5991+t6006-t6089+t6217+t6218+t6488+t6489+t6703+t6730+t6819-t6959-t6979+t7019+t7191+t7419+t7420+t7425+t7630+t8036+t8288+t8290+t8308-t8439-t8783-t8787+t8930+t8943+t9010+t9017+t9019-t9164+t9251+t9923+t9930+(t371.*(t689-t740))./4.0),t16116-t16218-t16246-t16276-t16377-q7d.*t16113+q5d.*t16150+xd.*(-t8786-t8793+t8848+t11052+t11062-t11847-t11974+t12684+t12708+t12795+t12810+t12855+t12863+t12875-t12969-t12975+t13003+t13004+t13061+t13075+t13076-t13096-t13100+t13188+t13469+t13473+t13648+t14509+t14510+t14618+t14625+t7.*t8.*(t4542-t6448).*1.17633784675e-2)+q6d.*(t8.*(-1.9409574471375e-3)+t16.*8.2699333773375e-3+t7.*t8.*3.849278081088e-2+t7.*t16.*9.03427466304e-3+t8.*t15.*9.3569097314605e-5-t15.*t16.*1.037589172186849e-4-t9.*t4474.*2.2652974317e-2+t17.*t4517.*2.2652974317e-2+(t17.*t4551)./2.0-(t9.*t4701)./2.0-t9.*t6397.*3.07985e-2+t17.*t6408.*3.07985e-2+(t4152.*t5365)./2.0+(t3489.*t6104)./2.0-(t16.*t41.*t3239)./2.0+(t8.*t15.*t3286)./2.0+(t16.*t45.*(t689-t740))./2.0)+q3d.*(t3775+t3786+t3787+t3920+t4029+t4037+t4091+t4106+t4132+t4182+t4207+t4240+t4247-t4891-t4926+t4961+t5036+t5146-t5372-t5398+t5421-t5678-t5816-t5817+t6004+t6023-t6086+t6705+t6722+t6754+t6842+t6882+t7285-t7298-t7325-t7333+t7431+t7447+t7678-t7716-t7729+t7762-t7766-t7770-t8247+t8489-t8744+t9018+t9027+t9191+t9282+t9287+t9461+t9479+t9493-t9516-t9517-t9646-t9671-t9683+t10135+t10136-(t9.*t323.*t5763)./4.0-(t17.*t323.*t5837)./4.0),t15782+t16153-t16168-t16199+t16231+t16234+q7d.*t15891+phid.*(-t4238+t4295-t4456+t4713+t4744+t4783+t4797+t4947+t5325+t5330+t5336+t5390+t5749+t5814+t6360+t6396+t7007+t7031+t7103+t7491+t7572+t7583+t8090+t8624+t8648+t8676+t8721+t11997+t13108-t13433+t13688-t13853+t14033+t14034+t14196+t14197+t14200+t14205+t14255+t14351+t14460+t14461+t14479+t14483+t14554+t14591+t14592+t14871-t14895-t15140+t15619+t15620+t15689+t15690+(t9.*(t578.*4.28e-4+t2566-t2597+t905.*(t71-t391)+t1021.*(t71-t391)))./4.0+t8.*(t210+t2107+t7423+t9121).*1.17633784675e-2+t17.*(-t2550+t2696+t2698+t11659+t8.*t11672+t147.*(t71-t391)).*1.13264871585e-2+t17.*(-t3823+t3970+t11861+t8.*t11864+t972.*(t71-t391)+t2777.*(t71-t391)).*1.539925e-2+t8.*(t71-t391).*5.187945860934245e-5+t16.*(t71-t391).*4.67845486573025e-5+(t2522.*(t689-t740))./4.0+(t16.*t3286.*(t71-t391))./4.0)-q6d.*(t8.*1.037589172186849e-4+t16.*9.3569097314605e-5+(t16.*t3286)./2.0+t8.*t3398+t8.*t3550-t9.*t3763.*2.2652974317e-2+t17.*t3767.*2.2652974317e-2-(t17.*t4432)./2.0+(t9.*t4499)./2.0-t9.*t5449.*3.07985e-2+t17.*t5448.*3.07985e-2-(t3455.*t5365)./2.0-(t3489.*(t2889-t2921))./2.0)+q1d.*(-t4238+t4295-t4456+t4713+t4744+t4783+t4797+t4947+t5325+t5330+t5336+t5390-t5666+t5675+t5749+t5814+t6360+t6396+t7007+t7031+t7103+t7491+t7572+t7583+t7859+t7884+t8090+t8624+t8648+t8676+t8721+t8929+t8935+t8936+t8947+t9148+t9180+t9653+t9689-t10006+t10009+t10011+t10121+t10130+t10329+t10497+t10518+t10522+t10756-t10808+t11280+t11285+t11454+t11992+t11996+(t9.*(t578.*4.28e-4+t2566-t2597+t905.*(t71-t391)+t1021.*(t71-t391)))./4.0+t17.*(-t3823+t3970+t5243+t9.*(t260+t468+t570+t2298).*7.35522e-1+t972.*(t71-t391)+t2777.*(t71-t391)).*1.539925e-2+t8.*(t71-t391).*5.187945860934245e-5+t16.*(t71-t391).*4.67845486573025e-5+(t2522.*(t689-t740))./4.0+t17.*(-t2550+t2696+t2698+t4771+t9.*(t260+t468+t570+t2298)+t147.*(t71-t391)).*1.13264871585e-2+(t16.*t3286.*(t71-t391))./4.0),q7d.*(t3355-t3398-t3536+t6133+t6524+(t17.*(t689-t740))./2.0),t11312-t15893-t16072-t16075-t16114+t16134+t16147+t16256+q3d.*(t3825+t3853-t3990-t4067+t4099+t4153+t4160+t4186+t4273+t4372+t4423-t5547+t5671+t6595+t6623-t6671-t6773-t7738-t7781+t7992-t8214+t8334+t8354+t8404-t9519-t9530+(t3239.*(t79-t358))./4.0+(t3280.*(t79-t358))./4.0+(t8640.*(t701-t775))./4.0),-q4d.*(t8863+t8883+t11354+t11371-t13105-t13266+t14530+t14539-t14599+t14684+t14687-t14797+(t5345.*(t10403+t9.*(t10158+t16.*(t4542-t6448)).*7.35522e-1))./4.0+(t7797.*(t10174+t9.*(t10158+t16.*(t4542-t6448))))./4.0)-phid.*t16296-q5d.*t16183-q3d.*t16200-q2d.*t16208-q1d.*t16221-q6d.*(t12494+t12498-t12750+(t12484.*(t701-t775))./4.0)+q7d.*(t10173.*(-3.127439544e-3)+t2772.*(t10158+t16.*(t4542-t6448))+t2775.*(t10158+t16.*(t4542-t6448))+t2778.*t10153),-q2d.*(t8350.*3.867742437e-3+t10735+t13312+t13522+t14948+t14954+t15093+t15095+t15099+t15109+t15295+t15304+t9.*(t16.*(t30.*(t2425-t2468)+t68.*(t2425-t2468))+t8.*(t7.*(t4650+t34.*(t2425-t2468))+t47.*(t2425-t2468))).*1.563719772e-3+t17.*(t4654+t15.*(t4650+t34.*(t2425-t2468))).*1.563719772e-3)-phid.*t16299-q5d.*t16186+q4d.*t16194-q3d.*t16203-q1d.*t16225-q6d.*(t12511+t12518-t12774+(t12500.*(t701-t775))./4.0)-q7d.*(t10218.*7.735484874e-3+t2772.*t12307+t2775.*t12307-t2769.*(t6452-t8229)),t16243+q6d.*t16255+q4d.*t16265+q3d.*t16270+q2d.*t16283+q5d.*(-t4652-t4658+t4757+t4825+t5253+t5305+t5766+t5791+t7139+t7199+t7204+t8632+t8677+t8904+t9266+t12008+t12014+t12018+t14555+t14872+t15553+t15555+t15600+t15602+t15607+t15609+t15671+t15672+t8.*t11672.*3.867742437e-3+t2963.*(t71-t391)+t3167.*(t71-t391)+t4080.*(t71-t391)+t4130.*(t71-t391))+q7d.*(t4666+t4722+t4980+t4981-t11672.*7.735484874e-3+t2769.*(t210+t2107+t7423+t9121)+t9.*(t71-t391).*1.672482661783778e-3+t2778.*(t426-t581)+t2772.*(t9166-t11658)+t2775.*(t9166-t11658))+xd.*(t10657+t10678+t12523+t12525-t13534-t13699-t16028+t16029+t16034-t16035+t16042+t16061+(t14185.*(t3418-t3879+t4324+t11855+t9.*(t71-t391).*4.5305948634e-2+t17.*(t426-t581).*7.35522e-1+t9.*(t9166-t11658).*7.35522e-1))./4.0+(t14280.*(t1987-t2621+t3452+t11654+t9.*(t71-t391).*6.1597e-2+t17.*(t426-t581)+t9.*(t9166-t11658)))./4.0)+yd.*(t10600+t10609+t12501+t12510-t13551-t13712+t16032+t16037+t16049+t16067+(t14299.*(t2497+t2680+t3516+t9.*(t210+t2107+t7423+t9121)+t17.*(t9166-t11658)))./4.0+(t14209.*(t3418-t3879+t4324+t11855+t9.*(t71-t391).*4.5305948634e-2+t17.*(t426-t581).*7.35522e-1+t9.*(t9166-t11658).*7.35522e-1))./4.0+(t14213.*(t3845+t3925+t4339+t9.*(t210+t2107+t7423+t9121).*7.35522e-1+t17.*(t9166-t11658).*7.35522e-1))./4.0+(t14297.*(t1987-t2621+t3452+t11654+t9.*(t71-t391).*6.1597e-2+t17.*(t426-t581)+t9.*(t9166-t11658)))./4.0)+q1d.*(t7826+t8162+t8296+t9175+t9204+t11976+t12459-t13211+t13214+t15017+t15219+t15823+t15825+t15827+t15828+t15859+t15861+t15863+t15866+t9.*(t8963+t7.*(t5026+t5.*(t2959-t2967))).*3.867742437e-3+t17.*(t8963+t7.*(t5026+t5.*(t2959-t2967))).*1.563719772e-3),t16136+t16280+xd.*(t10657+t10678+t12523+t12525-t13534-t13699+t15165+t15166+t15271+t15273+(t10149.*(t10403+t9.*(t10158+t16.*(t4542-t6448)).*7.35522e-1))./4.0+(t14185.*(t3418-t3879+t4324-t5228+t5802+t9.*(t71-t391).*4.5305948634e-2+t17.*(t426-t581).*7.35522e-1))./4.0+(t14280.*(t1987-t2621+t3452-t4730+t5359+t9.*(t71-t391).*6.1597e-2+t17.*(t426-t581)))./4.0+(t11470.*(t10174+t9.*(t10158+t16.*(t4542-t6448))))./4.0)+q6d.*t16146+q4d.*t16166+q3d.*t16173+q2d.*t16177+q7d.*(t4666+t4722-t4730.*7.735484874e-3+t4980+t4981+t2769.*t4618+t2772.*t5337+t2775.*t5337+t9.*(t71-t391).*1.672482661783778e-3+t2778.*(t426-t581))+q5d.*(-t4652-t4658+t4757+t4825+t5253+t5305+t5687-t5698+t5766+t5791+t7139+t7199+t7204+t8632+t8677+t8904+t9266+t10330+t10589+t10591+t10853+t10861+t10967+t10977+t11455+t11823+t11832+t9.*(t260+t468+t570+t2298).*3.867742437e-3+t17.*(t260+t468+t570+t2298).*1.563719772e-3+t2963.*(t71-t391)+t3167.*(t71-t391)+t4080.*(t71-t391)+t4130.*(t71-t391))+yd.*(t10600+t10609+t12501+t12510-t13551-t13712+t15181+t15182+t15289+t15293-t15358-t15476+(t14209.*(t3418-t3879+t4324-t5228+t5802+t9.*(t71-t391).*4.5305948634e-2+t17.*(t426-t581).*7.35522e-1))./4.0+(t14297.*(t1987-t2621+t3452-t4730+t5359+t9.*(t71-t391).*6.1597e-2+t17.*(t426-t581)))./4.0),t16124+t16179+t16210+t16282+yd.*(t8350.*3.867742437e-3+t10735+t13315+t13529+t14946+t14951+t15092+t15097+t15102+t15107+t15300+t15306+t9.*(t16.*(t30.*(t2425-t2468)+t68.*(t2425-t2468))+t8.*(t7.*(t4650+t34.*(t2425-t2468))+t47.*(t2425-t2468))).*1.563719772e-3+t17.*(t4654+t15.*(t4650+t34.*(t2425-t2468))).*1.563719772e-3)+q5d.*t16141-q6d.*(t4201+t4248-t4443-t4577+t4593+t4675+t4706+t4741+t4788-t5568+t5585+t6270+t6382+t7494+t7575+t8573+t8704+t8708+t8825+t9404+t9434+t9443+t9680+t9681+t10696+t10728+t10730+t9.*(t208-t427).*3.867742437e-3+t17.*(t208-t427).*1.563719772e-3)+q4d.*(t3995+t4013+t4190+t4197+t4271+t4313+t4437+t4467+t4543+t4560+t5106+t5166-t5688+t5906+t6001-t6439+t6487+t6491+t7633+t7758-t10457-t10565+t10573+t10755-t10760-t10844+t10845-t11160+t11236-t11240+(t5837.*(t395+t9.*(t48-t349)))./4.0+(t8477.*(-t2149+t2205+t693.*(t48-t349)+t784.*(t48-t349)))./4.0+(t5696.*(t3479-t3544+t2772.*(t48-t349)+t2775.*(t48-t349)))./4.0+(t15.*t16.*(-t2182+t2241+t696.*(t48-t349)+t891.*(t48-t349)))./4.0)+q3d.*(t1625.*1.563719772e-3+t4270-t4348-t4354-t4488+t4648-t4659+t5032+t5054-t5558+t5570+t5995+t6268+t6327+t6534+t6544+t6612+t7319+t7451+t7855+t7900+t9960+t10359+t10553+t11202+t11223+t11275+t11297+t11309+t11555+t11594+t11632+t11638+t9.*(t236-t451).*3.867742437e-3)+q7d.*(t389.*1.672482661783778e-3-t395.*5.48359106408232e-4+t718.*3.127439544e-3-t729.*7.735484874e-3-t3349.*7.735484874e-3+t2769.*t3268-t9.*(t48-t349).*5.48359106408232e-4-t17.*(t48-t349).*1.672482661783778e-3+t2772.*(t624-t3502)+t2775.*(t624-t3502)),-t16105+t16163-t16174+t16202+t16205-t16271+q7d.*(t49.*5.48359106408232e-4-t79.*1.672482661783778e-3+t352.*5.48359106408232e-4+t358.*1.672482661783778e-3-t531.*3.127439544e-3+t532.*7.735484874e-3-t615.*3.127439544e-3+t617.*7.735484874e-3-t778.*7.735484874e-3-t786.*3.127439544e-3)+q6d.*t16120-q5d.*t16127+q4d.*t16137,t16009-t16139-t16165+t16193+t16196-t16264+q2d.*(-t3995-t4013-t4190-t4197+t4291+t4306+t4448+t4462+t4520+t4539+t5127+t5140-t5688+t5906+t6001-t6439+t6487+t6491+t7633+t7758-t10457-t10565+t10573+t10755-t10760-t10844+t10845-t11160+t11236-t11240+(t5837.*(t395+t9.*(t48-t349)))./4.0+(t8477.*(-t2149+t2205+t693.*(t48-t349)+t784.*(t48-t349)))./4.0+(t5696.*(t3479-t3544+t2772.*(t48-t349)+t2775.*(t48-t349)))./4.0+(t15.*t16.*(-t2182+t2241+t696.*(t48-t349)+t891.*(t48-t349)))./4.0)-q7d.*(t33.*1.672482661783778e-3-t40.*5.48359106408232e-4+t41.*1.200936784896e-3-t45.*2.970426191616e-3+t67.*5.48359106408232e-4+t80.*1.672482661783778e-3-t452.*7.735484874e-3-t453.*3.127439544e-3+t16.*t41.*2.75214679872e-4-t16.*t45.*6.80722668912e-4)-q6d.*t16113+q5d.*t16119,-t14558+t16118+t16129+t16158+t16185+t16188+t16259+q7d.*(t8.*t9.*(-2.75214679872e-4)+t8.*t17.*6.80722668912e-4+t9.*t16.*5.48359106408232e-4+t16.*t17.*1.672482661783778e-3)+q2d.*(-t3674-t3725+t4277+t4347+t4353+t4442-t4449+t4817+t4823-t5008+t5022-t5031-t5053+t5313+t5380+t6316+t6414+t6419+t7516+t7587+t8265+t8818+t9453+t9582+t9596+t9758+t9762+t10065+t10069+t10721+t10803+t10811-t16.*t321.*2.454825983680473e-3)+q6d.*t15891,t15893+t16072+t16075+t16114+t16122+q2d.*(t4230+t4248-t4443-t4577+t4593+t4639+t4676+t4717+t4806-t5568+t5585+t6288+t6364+t7479+t7557+t8596+t8696+t8702+t8843+t9424+t9447+t9460+t9673+t9675+t10705+t10733+t10734+t9.*(t208-t427).*3.867742437e-3+t17.*(t208-t427).*1.563719772e-3)-q7d.*(t9.*1.672482661783778e-3-t17.*5.48359106408232e-4)+phid.*(-t4446-t4631-t4668-t4758+t4796+t5014+t5186+t5242+t5249+t5260+t7125+t7190+t8614+t8666+t9074+t9268-t13711+t13715+t14543+t14862+t15500+t15501+t15556+t15560+t15562+t15563+t15662+t15665+t9.*(t348-t525).*8.36241330891889e-4)+q1d.*(-t4446-t4631-t4668-t4758+t4796+t5014+t5186+t5242+t5249+t5260-t6377+t6390+t7125+t7190+t8614+t8666+t9074+t9268+t9882+t9885+t10307+t10601+t10606+t10707+t10708+t11438+t11702+t11703+t9.*(t348-t525).*8.36241330891889e-4)+q6d.*(t3355-t3398-t3536+t6133+t6524+(t17.*(t689-t740))./2.0),0.0],[10,10]);
